simulink model "Simulink_PID"  (R2021b)
settings: Solver=ode45  StartTime=0.0  StopTime=12  RelTol=1e-3
model workspace (MAT data in the model file):
  e = -5
settings Model: Creator=Shahday Bhai  LastModifiedBy=Shahday Bhai
settings SolverCC: AlgebraicLoopSolver=TrustRegion
settings DataIOCC: SaveFormat=StructureWithTime
settings OptimizationCC: LifeSpan=inf
settings DebuggingCC: SFExecutionAtInitializationDiag=none  SFMachineParentedDataDiag=warning  ArithmeticOperatorsInVariantConditions=warning
settings HardwareCC: ProdBitPerSizeT=32  ProdBitPerPtrDiffT=32  ProdWordSize=32  ProdHWDeviceType=Specified
settings SFSimCC: CustomCodeUndefinedFunction=UseInterfaceOnly
settings CodeAppCC: StateflowObjectComments=on

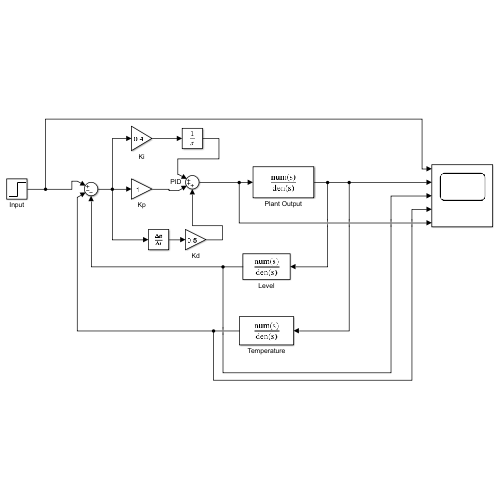
[thumbnail: Simulink's stored preview of the top-level diagram]
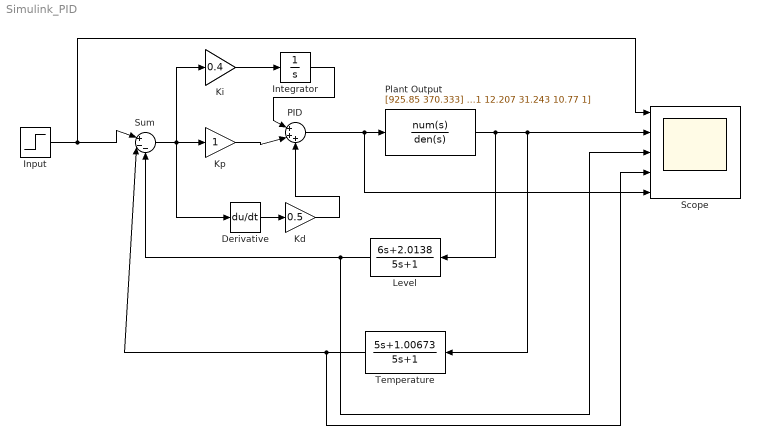
== system Simulink_PID ==
  Derivative : Derivative
  Input : Step  SampleTime=0
  Integrator : Integrator
  Kd : Gain  Gain=0.5
  Ki : Gain  Gain=0.4
  Kp : Gain
  Level : TransferFcn  Numerator=[6 2.0138]  Denominator=[5 1]
  PID : Sum  Inputs=|+++
  Plant Output : TransferFcn  Numerator=[925.85 370.333]  Denominator=[1.11 12.207 31.243 10.77 1]
  Scope : Scope  NumInputPorts=5
  Sum : Sum  Inputs=|+--
  Temperature : TransferFcn  Numerator=[5 1.00673]  Denominator=[5 1]
  wires:
  Input/1 -> Sum/1, Scope/1
  Sum/1 -> Derivative/1, Ki/1, Kp/1
  Ki/1 -> Integrator/1
  Integrator/1 -> PID/1
  Kp/1 -> PID/2
  Derivative/1 -> Kd/1
  Kd/1 -> PID/3
  Temperature/1 -> Scope/4, Sum/2
  PID/1 -> Scope/5, Plant Output/1
  Level/1 -> Scope/3, Sum/3
  Plant Output/1 -> Level/1, Temperature/1, Scope/2
